simulink model "top_model_rw_desatTest"  (R2017b)
settings: Solver=FixedStepAuto  StartTime=0.0  StopTime=30000  FixedStep=.2  RelTol=1e-3  EnableMultiTasking=on
model workspace: external: MATLAB File C:\Users\Justin\Documents\00 MEng Project\PAN_ADCS\initialization\simulink_workspace_init.m (data not in the file)
undefined symbols (not defined in the file): h_init, hdmax, hmax, IAU, Imp_max, Imp_min, init, K_F, Kd, km, Kp, L_F, m_follower, match_tol, muE, ontime_max, ontime_min, q_init, s, Thrust_max, Thrust_min, wbn_init
libraries: aerolibtransform2 x12, aerolibconvert2 x8, sharedtransform x8, hEemethod x8, aerolibgravity2 x6, aerolibutil x6, aerolibcelestial x4, vrlib x4
(part 4 of 5)

== system top_model_rw_desatTest/Controller1/Normal Mode Control System/compute attitude error ==
  quat : Inport
  quat_cmd : Inport  Port=2
  Demux : Demux
  Demux1 : Demux
  Mux : Mux  Inputs=3
  Mux1 : Mux  Inputs=2
  Mux2 : Mux  Inputs=3
  Mux3 : Mux  Inputs=2
  Selector : Selector  InputPortWidth=4  IndexOptions=Index vector (dialog)  Indices=4  OutputSizes=1
  Switch : Switch
  quat_multiply (relative quat) : Subsystem
  quat_multiply (relative quat)1 : Subsystem
  reverse : Gain  Gain=-1  SaturateOnIntegerOverflow=on  OutDataTypeStr=Inherit: Same as input  ParamDataTypeStr=Inherit: Same as input
  reverse1 : Gain  Gain=-1  SaturateOnIntegerOverflow=on  OutDataTypeStr=Inherit: Same as input  ParamDataTypeStr=Inherit: Same as input
  quat error : Outport
  wires:
  Demux/1 -> Mux/1
  Demux/2 -> Mux/2
  Demux/3 -> Mux/3
  Mux/1 -> reverse/1
  Mux1/1 -> quat_multiply (relative quat)/2(q_ab)
  Demux/4 -> Mux1/2
  reverse/1 -> Mux1/1
  Mux3/1 -> quat_multiply (relative quat)1/2(q_ab)
  Demux1/1 -> Mux2/1
  Demux1/2 -> Mux2/2
  Demux1/3 -> Mux2/3
  quat_cmd/1 -> Demux1/1, Demux/1
  Mux2/1 -> Mux3/1
  quat/1 -> quat_multiply (relative quat)1/1(q_bc), quat_multiply (relative quat)/1(q_bc)
  Demux1/4 -> reverse1/1
  reverse1/1 -> Mux3/2
  quat_multiply (relative quat)1/1(q_ac) -> Switch/3
  quat_multiply (relative quat)/1(q_ac) -> Selector/1, Switch/1
  Switch/1 -> quat error/1
  Selector/1 -> Switch/2

== system top_model_rw_desatTest/Controller1/Propulsion/Enabled Subsystem ==
  In1 : Inport
  Enable : EnablePort
  Out1 : Outport
  wires:
  In1/1 -> Out1/1

== system top_model_rw_desatTest/Controller1/Propulsion/Subsystem ==
  hit : Inport
  ontime : Inport  Port=2
  "Thrust_vec " : Inport  Port=3
  Activation : Subsystem
  Constant1 : Constant  Value=[0;0;0]
  Subsystem : Subsystem
  Switch : Switch  Criteria=u2 > Threshold
  imp_cmd : Outport
  wires:
  Constant1/1 -> Switch/3
  ontime/1 -> Activation/2(T_maneuver)
  Subsystem/1(value) -> Switch/2
  "Thrust_vec "/1 -> Switch/1
  hit/1 -> Subsystem/1(input), Activation/1(hit)
  Activation/1(man_end) -> Subsystem/2(overwrite trigger)
  Switch/1 -> imp_cmd/1

== system top_model_rw_desatTest/Controller1/Propulsion/Subsystem1 ==
  input : Inport
  overwrite trigger : Inport  Port=2
  Data Store Memory : DataStoreMemory  DataStoreName=Mem  ShowAdditionalParam=off
  Data Store Read : DataStoreRead  DataStoreName=Mem  SampleTime=[0,0]  DataStoreElements=Mem
  Data Store Write : DataStoreWrite  DataStoreName=Mem  SampleTime=[0,0]  DataStoreElements=Mem
  Switch : Switch  Criteria=u2 > Threshold
  value : Outport
  wires:
  input/1 -> Switch/1
  Switch/1 -> value/1, Data Store Write/1
  Data Store Read/1 -> Switch/3
  overwrite trigger/1 -> Switch/2

== system top_model_rw_desatTest/Controller1/quat to DCM/Subsystem ==
  In1 : Inport
  3x3 : Reshape  OutputDimensionality=Customize  OutputDimensions=[3,3]
  Demux : Demux  Outputs=3
  Gain : Gain  Gain=-1  SaturateOnIntegerOverflow=on  OutDataTypeStr=Inherit: Same as input  ParamDataTypeStr=Inherit: Same as input
  Gain1 : Gain  Gain=-1  SaturateOnIntegerOverflow=on  OutDataTypeStr=Inherit: Same as input  ParamDataTypeStr=Inherit: Same as input
  Gain2 : Gain  Gain=-1  SaturateOnIntegerOverflow=on  OutDataTypeStr=Inherit: Same as input  ParamDataTypeStr=Inherit: Same as input
  Mux : Mux  Inputs=9
  "diag 0 " : Constant  Value=0
  Out1 : Outport
  wires:
  In1/1 -> Demux/1
  3x3/1 -> Out1/1
  "diag 0 "/1 -> Mux/1, Mux/5, Mux/9
  Mux/1 -> 3x3/1
  Demux/3 -> Mux/2, Gain1/1
  Gain/1 -> Mux/3
  Demux/2 -> Gain/1, Mux/7
  Gain1/1 -> Mux/4
  Demux/1 -> Mux/6, Gain2/1
  Gain2/1 -> Mux/8

== system top_model_rw_desatTest/FWR_Plant/Quaternion Integration/q_normalize ==
  q_in : Inport  PortDimensions=4
  Dot Product : DotProduct  InputSameDT=on  OutDataTypeStr=Inherit: Inherit via internal rule
  Math Function : Math  Operator=sqrt  SaturateOnIntegerOverflow=on
  Product : Product  Inputs=*/  SaturateOnIntegerOverflow=on  InputSameDT=on  OutDataTypeStr=Inherit: Same as first input
  q_out : Outport
  wires:
  q_in/1 -> Dot Product/1, Dot Product/2, Product/1
  Dot Product/1 -> Math Function/1
  Math Function/1 -> Product/2
  Product/1 -> q_out/1

== system top_model_rw_desatTest/FWR_Plant/Quaternion Integration/qderiv ==
  w : Inport
  q : Inport  Port=2
  Mux : Mux  Inputs=2
  Mux1 : Mux
  qd1 : Fcn  Expr=(u(7)*u(1)-u(6)*u(2)+u(5)*u(3))/2
  qd2 : Fcn  Expr=(u(6)*u(1)+u(7)*u(2)-u(4)*u(3))/2
  qd3 : Fcn  Expr=(-u(5)*u(1)+u(4)*u(2)+u(7)*u(3))/2
  qd4 : Fcn  Expr=(-u(4)*u(1)-u(5)*u(2)-u(6)*u(3))/2
  qd : Outport
  wires:
  w/1 -> Mux/1
  q/1 -> Mux/2
  Mux/1 -> qd3/1, qd4/1, qd1/1, qd2/1
  qd1/1 -> Mux1/1
  qd2/1 -> Mux1/2
  qd3/1 -> Mux1/3
  qd4/1 -> Mux1/4
  Mux1/1 -> qd/1

== system top_model_rw_desatTest/FWR_Sensor Model/quat to DCM/Subsystem ==
  In1 : Inport
  3x3 : Reshape  OutputDimensionality=Customize  OutputDimensions=[3,3]
  Demux : Demux  Outputs=3
  Gain : Gain  Gain=-1  SaturateOnIntegerOverflow=on  OutDataTypeStr=Inherit: Same as input  ParamDataTypeStr=Inherit: Same as input
  Gain1 : Gain  Gain=-1  SaturateOnIntegerOverflow=on  OutDataTypeStr=Inherit: Same as input  ParamDataTypeStr=Inherit: Same as input
  Gain2 : Gain  Gain=-1  SaturateOnIntegerOverflow=on  OutDataTypeStr=Inherit: Same as input  ParamDataTypeStr=Inherit: Same as input
  Mux : Mux  Inputs=9
  "diag 0 " : Constant  Value=0
  Out1 : Outport
  wires:
  In1/1 -> Demux/1
  3x3/1 -> Out1/1
  "diag 0 "/1 -> Mux/1, Mux/5, Mux/9
  Mux/1 -> 3x3/1
  Demux/3 -> Mux/2, Gain1/1
  Gain/1 -> Mux/3
  Demux/2 -> Gain/1, Mux/7
  Gain1/1 -> Mux/4
  Demux/1 -> Mux/6, Gain2/1
  Gain2/1 -> Mux/8

== system top_model_rw_desatTest/GNC/Follower Maneuver/Optimal Latitude Calc ==
  "r " : Inport
  "v " : Inport  Port=2
  muE : Inport  Port=3
  x_tgt : Inport  Port=4
  x_f : Inport  Port=5
  Update Trigger : Inport  Port=6
  Constant : Constant  Value=K_F
  Constant1 : Constant  Value=L_F
  Enabled Subsystem : Subsystem  TreatAsAtomicUnit=on
  dV_opt : Outport
  long_opt : Outport  Port=2
  pos_opt : Outport  Port=3
  wires:
  Enabled Subsystem/2(long_opt) -> long_opt/1
  "r "/1 -> Enabled Subsystem/1(r)
  "v "/1 -> Enabled Subsystem/2(v)
  muE/1 -> Enabled Subsystem/7("muE ")
  x_tgt/1 -> Enabled Subsystem/3(x_tgt)
  x_f/1 -> Enabled Subsystem/4(x_f)
  Constant/1 -> Enabled Subsystem/5(K)
  Constant1/1 -> Enabled Subsystem/6(L)
  Enabled Subsystem/1(dV_opt) -> dV_opt/1
  Enabled Subsystem/3(pos_opt) -> pos_opt/1
  Update Trigger/1 -> Enabled Subsystem/Enable

== system top_model_rw_desatTest/LDR_Plant/Quaternion Integration/q_normalize ==
  q_in : Inport  PortDimensions=4
  Dot Product : DotProduct  InputSameDT=on  OutDataTypeStr=Inherit: Inherit via internal rule
  Math Function : Math  Operator=sqrt  SaturateOnIntegerOverflow=on
  Product : Product  Inputs=*/  SaturateOnIntegerOverflow=on  InputSameDT=on  OutDataTypeStr=Inherit: Same as first input
  q_out : Outport
  wires:
  q_in/1 -> Dot Product/1, Dot Product/2, Product/1
  Dot Product/1 -> Math Function/1
  Math Function/1 -> Product/2
  Product/1 -> q_out/1

== system top_model_rw_desatTest/LDR_Plant/Quaternion Integration/qderiv ==
  w : Inport
  q : Inport  Port=2
  Mux : Mux  Inputs=2
  Mux1 : Mux
  qd1 : Fcn  Expr=(u(7)*u(1)-u(6)*u(2)+u(5)*u(3))/2
  qd2 : Fcn  Expr=(u(6)*u(1)+u(7)*u(2)-u(4)*u(3))/2
  qd3 : Fcn  Expr=(-u(5)*u(1)+u(4)*u(2)+u(7)*u(3))/2
  qd4 : Fcn  Expr=(-u(4)*u(1)-u(5)*u(2)-u(6)*u(3))/2
  qd : Outport
  wires:
  w/1 -> Mux/1
  q/1 -> Mux/2
  Mux/1 -> qd3/1, qd4/1, qd1/1, qd2/1
  qd1/1 -> Mux1/1
  qd2/1 -> Mux1/2
  qd3/1 -> Mux1/3
  qd4/1 -> Mux1/4
  Mux1/1 -> qd/1

== system top_model_rw_desatTest/LDR_Sensor Model/quat to DCM/Subsystem ==
  In1 : Inport
  3x3 : Reshape  OutputDimensionality=Customize  OutputDimensions=[3,3]
  Demux : Demux  Outputs=3
  Gain : Gain  Gain=-1  SaturateOnIntegerOverflow=on  OutDataTypeStr=Inherit: Same as input  ParamDataTypeStr=Inherit: Same as input
  Gain1 : Gain  Gain=-1  SaturateOnIntegerOverflow=on  OutDataTypeStr=Inherit: Same as input  ParamDataTypeStr=Inherit: Same as input
  Gain2 : Gain  Gain=-1  SaturateOnIntegerOverflow=on  OutDataTypeStr=Inherit: Same as input  ParamDataTypeStr=Inherit: Same as input
  Mux : Mux  Inputs=9
  "diag 0 " : Constant  Value=0
  Out1 : Outport
  wires:
  In1/1 -> Demux/1
  3x3/1 -> Out1/1
  "diag 0 "/1 -> Mux/1, Mux/5, Mux/9
  Mux/1 -> 3x3/1
  Demux/3 -> Mux/2, Gain1/1
  Gain/1 -> Mux/3
  Demux/2 -> Gain/1, Mux/7
  Gain1/1 -> Mux/4
  Demux/1 -> Mux/6, Gain2/1
  Gain2/1 -> Mux/8

== system top_model_rw_desatTest/Actuator Model/Rigid Body with Momentum Actuators and energy dissipation/quat to DCM/Subsystem ==
  In1 : Inport
  3x3 : Reshape  OutputDimensionality=Customize  OutputDimensions=[3,3]
  Demux : Demux  Outputs=3
  Gain : Gain  Gain=-1  SaturateOnIntegerOverflow=on  OutDataTypeStr=Inherit: Same as input  ParamDataTypeStr=Inherit: Same as input
  Gain1 : Gain  Gain=-1  SaturateOnIntegerOverflow=on  OutDataTypeStr=Inherit: Same as input  ParamDataTypeStr=Inherit: Same as input
  Gain2 : Gain  Gain=-1  SaturateOnIntegerOverflow=on  OutDataTypeStr=Inherit: Same as input  ParamDataTypeStr=Inherit: Same as input
  Mux : Mux  Inputs=9
  "diag 0 " : Constant  Value=0
  Out1 : Outport
  wires:
  Gain2/1 -> Mux/8
  Demux/1 -> Gain2/1, Mux/6
  Gain1/1 -> Mux/4
  Demux/2 -> Mux/7, Gain/1
  Gain/1 -> Mux/3
  Demux/3 -> Gain1/1, Mux/2
  Mux/1 -> 3x3/1
  "diag 0 "/1 -> Mux/9, Mux/5, Mux/1
  3x3/1 -> Out1/1
  In1/1 -> Demux/1

== system top_model_rw_desatTest/Actuator Model/Rigid Body with Momentum Actuators and energy dissipation/quat to DCM1/Subsystem ==
  In1 : Inport
  3x3 : Reshape  OutputDimensionality=Customize  OutputDimensions=[3,3]
  Demux : Demux  Outputs=3
  Gain : Gain  Gain=-1  SaturateOnIntegerOverflow=on  OutDataTypeStr=Inherit: Same as input  ParamDataTypeStr=Inherit: Same as input
  Gain1 : Gain  Gain=-1  SaturateOnIntegerOverflow=on  OutDataTypeStr=Inherit: Same as input  ParamDataTypeStr=Inherit: Same as input
  Gain2 : Gain  Gain=-1  SaturateOnIntegerOverflow=on  OutDataTypeStr=Inherit: Same as input  ParamDataTypeStr=Inherit: Same as input
  Mux : Mux  Inputs=9
  "diag 0 " : Constant  Value=0
  Out1 : Outport
  wires:
  Gain2/1 -> Mux/8
  Demux/1 -> Gain2/1, Mux/6
  Gain1/1 -> Mux/4
  Demux/2 -> Mux/7, Gain/1
  Gain/1 -> Mux/3
  Demux/3 -> Gain1/1, Mux/2
  Mux/1 -> 3x3/1
  "diag 0 "/1 -> Mux/9, Mux/5, Mux/1
  3x3/1 -> Out1/1
  In1/1 -> Demux/1

== system top_model_rw_desatTest/Actuator Model1/Rigid Body with Momentum Actuators and energy dissipation/quat to DCM/Subsystem ==
  In1 : Inport
  3x3 : Reshape  OutputDimensionality=Customize  OutputDimensions=[3,3]
  Demux : Demux  Outputs=3
  Gain : Gain  Gain=-1  SaturateOnIntegerOverflow=on  OutDataTypeStr=Inherit: Same as input  ParamDataTypeStr=Inherit: Same as input
  Gain1 : Gain  Gain=-1  SaturateOnIntegerOverflow=on  OutDataTypeStr=Inherit: Same as input  ParamDataTypeStr=Inherit: Same as input
  Gain2 : Gain  Gain=-1  SaturateOnIntegerOverflow=on  OutDataTypeStr=Inherit: Same as input  ParamDataTypeStr=Inherit: Same as input
  Mux : Mux  Inputs=9
  "diag 0 " : Constant  Value=0
  Out1 : Outport
  wires:
  Gain2/1 -> Mux/8
  Demux/1 -> Gain2/1, Mux/6
  Gain1/1 -> Mux/4
  Demux/2 -> Mux/7, Gain/1
  Gain/1 -> Mux/3
  Demux/3 -> Gain1/1, Mux/2
  Mux/1 -> 3x3/1
  "diag 0 "/1 -> Mux/9, Mux/5, Mux/1
  3x3/1 -> Out1/1
  In1/1 -> Demux/1

== system top_model_rw_desatTest/Actuator Model1/Rigid Body with Momentum Actuators and energy dissipation/quat to DCM1/Subsystem ==
  In1 : Inport
  3x3 : Reshape  OutputDimensionality=Customize  OutputDimensions=[3,3]
  Demux : Demux  Outputs=3
  Gain : Gain  Gain=-1  SaturateOnIntegerOverflow=on  OutDataTypeStr=Inherit: Same as input  ParamDataTypeStr=Inherit: Same as input
  Gain1 : Gain  Gain=-1  SaturateOnIntegerOverflow=on  OutDataTypeStr=Inherit: Same as input  ParamDataTypeStr=Inherit: Same as input
  Gain2 : Gain  Gain=-1  SaturateOnIntegerOverflow=on  OutDataTypeStr=Inherit: Same as input  ParamDataTypeStr=Inherit: Same as input
  Mux : Mux  Inputs=9
  "diag 0 " : Constant  Value=0
  Out1 : Outport
  wires:
  Gain2/1 -> Mux/8
  Demux/1 -> Gain2/1, Mux/6
  Gain1/1 -> Mux/4
  Demux/2 -> Mux/7, Gain/1
  Gain/1 -> Mux/3
  Demux/3 -> Gain1/1, Mux/2
  Mux/1 -> 3x3/1
  "diag 0 "/1 -> Mux/9, Mux/5, Mux/1
  3x3/1 -> Out1/1
  In1/1 -> Demux/1

== system top_model_rw_desatTest/Attitude Determination and Desired Attitude/Attitude Determination/Generate reference vectors from Ephemeris and Magnetic Field Model/DecimalYearIncrement ==
  note: day
  clock_sec : Inport
  Add : Sum
  Constant : Constant  Value=init.year
  Constant1 : Constant  Value=init.month
  Constant2 : Constant  Value=init.day
  Constant3 : Constant  Value=init.hour
  Constant4 : Constant  Value=init.min
  Constant5 : Constant  Value=init.min
  Divide : Product  Inputs=*/
  MATLAB Function : MATLAB Function  TreatAsAtomicUnit=on
  Product2 : Product  Inputs=*/
  day2decimalYear : Constant  Value=365
  sec2day : Constant  Value=86400
  DecimalYear : Outport
  wires:
  Product2/1 -> Divide/1
  sec2day/1 -> Product2/2
  Add/1 -> DecimalYear/1
  Constant3/1 -> MATLAB Function/4(hour)
  day2decimalYear/1 -> Divide/2
  Divide/1 -> Add/1
  MATLAB Function/1(DecimalYear) -> Add/2
  Constant1/1 -> MATLAB Function/2(month)
  Constant/1 -> MATLAB Function/1(year)
  Constant4/1 -> MATLAB Function/5(minute)
  Constant5/1 -> MATLAB Function/6(second)
  clock_sec/1 -> Product2/1
  Constant2/1 -> MATLAB Function/3(day)

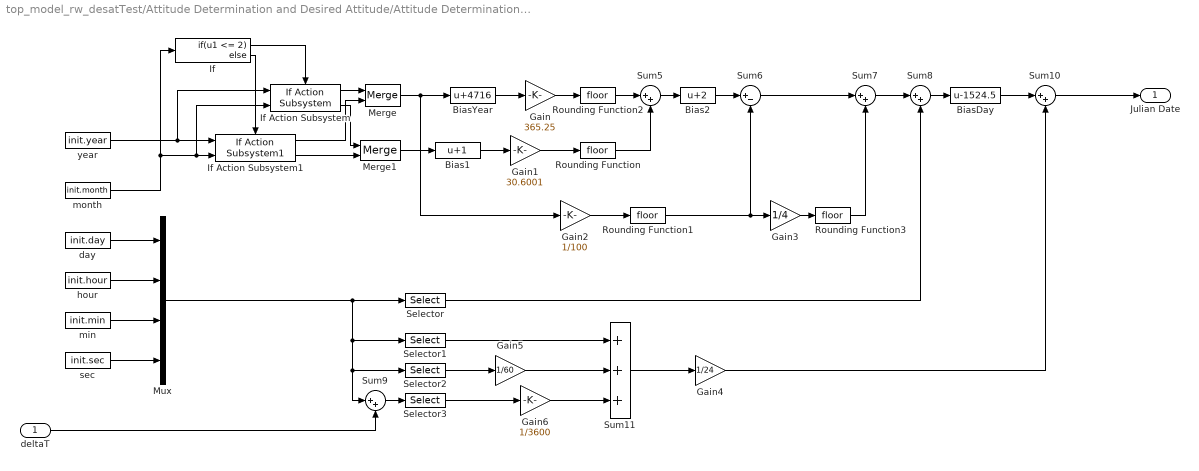
== system top_model_rw_desatTest/Attitude Determination and Desired Attitude/Attitude Determination/Generate reference vectors from Ephemeris and Magnetic Field Model/Julian Date ==
  deltaT : Inport  OutMin=0  PortDimensions=1
  Bias1 : Bias  Bias=1
  Bias2 : Bias  Bias=2
  BiasDay : Bias  Bias=-1524.5
  BiasYear : Bias  Bias=4716
  Gain : Gain  Gain=365.25
  Gain1 : Gain  Gain=30.6001
  Gain2 : Gain  Gain=1/100
  Gain3 : Gain  Gain=1/4
  Gain4 : Gain  Gain=1/24
  Gain5 : Gain  Gain=1/60
  Gain6 : Gain  Gain=1/3600
  If : If  IfExpression=u1 <= 2
  If Action Subsystem : aerolibconvert2/Julian Date Conversion/If Action Subsystem
      settings: SourceProductName=Aerospace Blockset  SourceProductBaseCode=AE
  If Action Subsystem1 : aerolibconvert2/Julian Date Conversion/If Action Subsystem1
      settings: SourceProductName=Aerospace Blockset  SourceProductBaseCode=AE
  Merge : Merge
  Merge1 : Merge
  Mux : Mux
  Rounding Function{,1..3} (4 alike) : Rounding
  Selector : Selector  InputPortWidth=4  IndexOptions=Index vector (dialog)  Indices=[1]  OutputSizes=1
  Selector1 : Selector  InputPortWidth=4  IndexOptions=Index vector (dialog)  Indices=[2]  OutputSizes=1
  Selector2 : Selector  InputPortWidth=4  IndexOptions=Index vector (dialog)  Indices=[3]  OutputSizes=1
  Selector3 : Selector  InputPortWidth=4  IndexOptions=Index vector (dialog)  Indices=[4]  OutputSizes=1
  Sum{5,7..10} (5 alike) : Sum  Inputs=|++
  Sum11 : Sum  Inputs=+++
  Sum6 : Sum  Inputs=|+-
  day : Constant  Value=init.day
  hour : Constant  Value=init.hour
  min : Constant  Value=init.min
  month : Constant  Value=init.month
  sec : Constant  Value=init.sec
  year : Constant  Value=init.year
  Julian Date : Outport
  wires:
  If Action Subsystem/1 -> Merge/1
  If/2 -> If Action Subsystem1/Action
  year/1 -> If Action Subsystem/1, If Action Subsystem1/1
  If/1 -> If Action Subsystem/Action
  If Action Subsystem/2 -> Merge1/1
  Rounding Function3/1 -> Sum7/2
  deltaT/1 -> Sum9/2
  day/1 -> Mux/1
  Merge1/1 -> Bias1/1
  Gain/1 -> Rounding Function2/1
  Gain2/1 -> Rounding Function1/1
  Merge/1 -> Gain2/1, BiasYear/1
  Selector3/1 -> Gain6/1
  Sum6/1 -> Sum7/1
  Gain5/1 -> Sum11/2
  BiasYear/1 -> Gain/1
  Selector2/1 -> Gain5/1
  Gain6/1 -> Sum11/3
  Sum11/1 -> Gain4/1
  Gain3/1 -> Rounding Function3/1
  Selector1/1 -> Sum11/1
  If Action Subsystem1/1 -> Merge/2
  Sum7/1 -> Sum8/1
  Mux/1 -> Selector1/1, Sum9/1, Selector2/1, Selector/1
  Sum10/1 -> Julian Date/1
  Selector/1 -> Sum8/2
  Bias1/1 -> Gain1/1
  sec/1 -> Mux/4
  If Action Subsystem1/2 -> Merge1/2
  Sum5/1 -> Bias2/1
  BiasDay/1 -> Sum10/1
  Gain1/1 -> Rounding Function/1
  Rounding Function1/1 -> Gain3/1, Sum6/2
  Bias2/1 -> Sum6/1
  Sum8/1 -> BiasDay/1
  Rounding Function2/1 -> Sum5/1
  Rounding Function/1 -> Sum5/2
  month/1 -> If Action Subsystem/2, If Action Subsystem1/2, If/1
  min/1 -> Mux/3
  hour/1 -> Mux/2
  Gain4/1 -> Sum10/2
  Sum9/1 -> Selector3/1

== system top_model_rw_desatTest/Attitude Determination and Desired Attitude/Position and Velocity to Desired Attitude in Quat/CreateDCM_be/normalize ==
  r : Inport
  Dot Product : DotProduct  InputSameDT=on  OutDataTypeStr=Inherit: Inherit via internal rule
  Math Function : Math  Operator=sqrt  SaturateOnIntegerOverflow=on
  Product : Product  Inputs=*/  SaturateOnIntegerOverflow=on  InputSameDT=on  OutDataTypeStr=Inherit: Same as first input
  r_hat : Outport
  wires:
  r/1 -> Dot Product/1, Dot Product/2, Product/1
  Dot Product/1 -> Math Function/1
  Math Function/1 -> Product/2
  Product/1 -> r_hat/1

== system top_model_rw_desatTest/Attitude Determination and Desired Attitude/Position and Velocity to Desired Attitude in Quat/CreateDCM_be/normalize2 ==
  v : Inport
  Dot Product : DotProduct  InputSameDT=on  OutDataTypeStr=Inherit: Inherit via internal rule
  Math Function : Math  Operator=sqrt  SaturateOnIntegerOverflow=on
  Product : Product  Inputs=*/  SaturateOnIntegerOverflow=on  InputSameDT=on  OutDataTypeStr=Inherit: Same as first input
  v_hat : Outport
  wires:
  v/1 -> Dot Product/1, Dot Product/2, Product/1
  Dot Product/1 -> Math Function/1
  Math Function/1 -> Product/2
  Product/1 -> v_hat/1

== system top_model_rw_desatTest/Attitude Determination and Desired Attitude/Position and Velocity to Desired Attitude in Quat/quat to DCM/Subsystem ==
  In1 : Inport
  3x3 : Reshape  OutputDimensionality=Customize  OutputDimensions=[3,3]
  Demux : Demux  Outputs=3
  Gain : Gain  Gain=-1  SaturateOnIntegerOverflow=on  OutDataTypeStr=Inherit: Same as input  ParamDataTypeStr=Inherit: Same as input
  Gain1 : Gain  Gain=-1  SaturateOnIntegerOverflow=on  OutDataTypeStr=Inherit: Same as input  ParamDataTypeStr=Inherit: Same as input
  Gain2 : Gain  Gain=-1  SaturateOnIntegerOverflow=on  OutDataTypeStr=Inherit: Same as input  ParamDataTypeStr=Inherit: Same as input
  Mux : Mux  Inputs=9
  "diag 0 " : Constant  Value=0
  Out1 : Outport
  wires:
  Gain2/1 -> Mux/8
  Demux/1 -> Gain2/1, Mux/6
  Gain1/1 -> Mux/4
  Demux/2 -> Mux/7, Gain/1
  Gain/1 -> Mux/3
  Demux/3 -> Gain1/1, Mux/2
  Mux/1 -> 3x3/1
  "diag 0 "/1 -> Mux/9, Mux/5, Mux/1
  3x3/1 -> Out1/1
  In1/1 -> Demux/1

== system top_model_rw_desatTest/Attitude Determination and Desired Attitude1/Attitude Determination/Generate reference vectors from Ephemeris and Magnetic Field Model/DecimalYearIncrement ==
  note: day
  clock_sec : Inport
  Add : Sum
  Constant : Constant  Value=init.year
  Constant1 : Constant  Value=init.month
  Constant2 : Constant  Value=init.day
  Constant3 : Constant  Value=init.hour
  Constant4 : Constant  Value=init.min
  Constant5 : Constant  Value=init.min
  Divide : Product  Inputs=*/
  MATLAB Function : MATLAB Function  TreatAsAtomicUnit=on
  Product2 : Product  Inputs=*/
  day2decimalYear : Constant  Value=365
  sec2day : Constant  Value=86400
  DecimalYear : Outport
  wires:
  Product2/1 -> Divide/1
  sec2day/1 -> Product2/2
  Add/1 -> DecimalYear/1
  Constant3/1 -> MATLAB Function/4(hour)
  day2decimalYear/1 -> Divide/2
  Divide/1 -> Add/1
  MATLAB Function/1(DecimalYear) -> Add/2
  Constant1/1 -> MATLAB Function/2(month)
  Constant/1 -> MATLAB Function/1(year)
  Constant4/1 -> MATLAB Function/5(minute)
  Constant5/1 -> MATLAB Function/6(second)
  clock_sec/1 -> Product2/1
  Constant2/1 -> MATLAB Function/3(day)

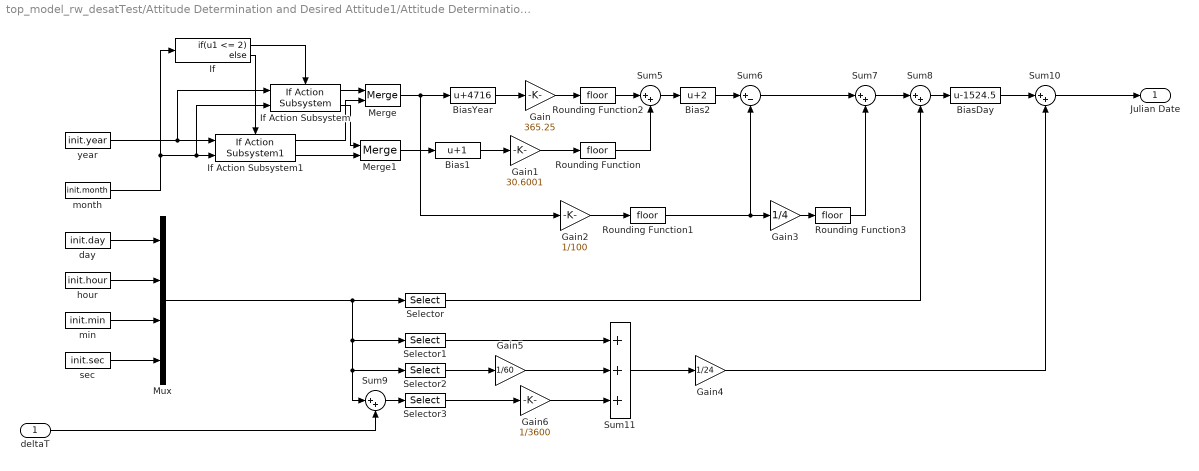
== system top_model_rw_desatTest/Attitude Determination and Desired Attitude1/Attitude Determination/Generate reference vectors from Ephemeris and Magnetic Field Model/Julian Date ==
  deltaT : Inport  OutMin=0  PortDimensions=1
  Bias1 : Bias  Bias=1
  Bias2 : Bias  Bias=2
  BiasDay : Bias  Bias=-1524.5
  BiasYear : Bias  Bias=4716
  Gain : Gain  Gain=365.25
  Gain1 : Gain  Gain=30.6001
  Gain2 : Gain  Gain=1/100
  Gain3 : Gain  Gain=1/4
  Gain4 : Gain  Gain=1/24
  Gain5 : Gain  Gain=1/60
  Gain6 : Gain  Gain=1/3600
  If : If  IfExpression=u1 <= 2
  If Action Subsystem : aerolibconvert2/Julian Date Conversion/If Action Subsystem
      settings: SourceProductName=Aerospace Blockset  SourceProductBaseCode=AE
  If Action Subsystem1 : aerolibconvert2/Julian Date Conversion/If Action Subsystem1
      settings: SourceProductName=Aerospace Blockset  SourceProductBaseCode=AE
  Merge : Merge
  Merge1 : Merge
  Mux : Mux
  Rounding Function{,1..3} (4 alike) : Rounding
  Selector : Selector  InputPortWidth=4  IndexOptions=Index vector (dialog)  Indices=[1]  OutputSizes=1
  Selector1 : Selector  InputPortWidth=4  IndexOptions=Index vector (dialog)  Indices=[2]  OutputSizes=1
  Selector2 : Selector  InputPortWidth=4  IndexOptions=Index vector (dialog)  Indices=[3]  OutputSizes=1
  Selector3 : Selector  InputPortWidth=4  IndexOptions=Index vector (dialog)  Indices=[4]  OutputSizes=1
  Sum{5,7..10} (5 alike) : Sum  Inputs=|++
  Sum11 : Sum  Inputs=+++
  Sum6 : Sum  Inputs=|+-
  day : Constant  Value=init.day
  hour : Constant  Value=init.hour
  min : Constant  Value=init.min
  month : Constant  Value=init.month
  sec : Constant  Value=init.sec
  year : Constant  Value=init.year
  Julian Date : Outport
  wires:
  If Action Subsystem/1 -> Merge/1
  If/2 -> If Action Subsystem1/Action
  year/1 -> If Action Subsystem/1, If Action Subsystem1/1
  If/1 -> If Action Subsystem/Action
  If Action Subsystem/2 -> Merge1/1
  Rounding Function3/1 -> Sum7/2
  deltaT/1 -> Sum9/2
  day/1 -> Mux/1
  Merge1/1 -> Bias1/1
  Gain/1 -> Rounding Function2/1
  Gain2/1 -> Rounding Function1/1
  Merge/1 -> Gain2/1, BiasYear/1
  Selector3/1 -> Gain6/1
  Sum6/1 -> Sum7/1
  Gain5/1 -> Sum11/2
  BiasYear/1 -> Gain/1
  Selector2/1 -> Gain5/1
  Gain6/1 -> Sum11/3
  Sum11/1 -> Gain4/1
  Gain3/1 -> Rounding Function3/1
  Selector1/1 -> Sum11/1
  If Action Subsystem1/1 -> Merge/2
  Sum7/1 -> Sum8/1
  Mux/1 -> Selector1/1, Sum9/1, Selector2/1, Selector/1
  Sum10/1 -> Julian Date/1
  Selector/1 -> Sum8/2
  Bias1/1 -> Gain1/1
  sec/1 -> Mux/4
  If Action Subsystem1/2 -> Merge1/2
  Sum5/1 -> Bias2/1
  BiasDay/1 -> Sum10/1
  Gain1/1 -> Rounding Function/1
  Rounding Function1/1 -> Gain3/1, Sum6/2
  Bias2/1 -> Sum6/1
  Sum8/1 -> BiasDay/1
  Rounding Function2/1 -> Sum5/1
  Rounding Function/1 -> Sum5/2
  month/1 -> If Action Subsystem/2, If Action Subsystem1/2, If/1
  min/1 -> Mux/3
  hour/1 -> Mux/2
  Gain4/1 -> Sum10/2
  Sum9/1 -> Selector3/1

== system top_model_rw_desatTest/Attitude Determination and Desired Attitude1/Position and Velocity to Desired Attitude in Quat/CreateDCM_be/normalize ==
  r : Inport
  Dot Product : DotProduct  InputSameDT=on  OutDataTypeStr=Inherit: Inherit via internal rule
  Math Function : Math  Operator=sqrt  SaturateOnIntegerOverflow=on
  Product : Product  Inputs=*/  SaturateOnIntegerOverflow=on  InputSameDT=on  OutDataTypeStr=Inherit: Same as first input
  r_hat : Outport
  wires:
  r/1 -> Dot Product/1, Dot Product/2, Product/1
  Dot Product/1 -> Math Function/1
  Math Function/1 -> Product/2
  Product/1 -> r_hat/1

== system top_model_rw_desatTest/Attitude Determination and Desired Attitude1/Position and Velocity to Desired Attitude in Quat/CreateDCM_be/normalize2 ==
  v : Inport
  Dot Product : DotProduct  InputSameDT=on  OutDataTypeStr=Inherit: Inherit via internal rule
  Math Function : Math  Operator=sqrt  SaturateOnIntegerOverflow=on
  Product : Product  Inputs=*/  SaturateOnIntegerOverflow=on  InputSameDT=on  OutDataTypeStr=Inherit: Same as first input
  v_hat : Outport
  wires:
  v/1 -> Dot Product/1, Dot Product/2, Product/1
  Dot Product/1 -> Math Function/1
  Math Function/1 -> Product/2
  Product/1 -> v_hat/1

== system top_model_rw_desatTest/Attitude Determination and Desired Attitude1/Position and Velocity to Desired Attitude in Quat/quat to DCM/Subsystem ==
  In1 : Inport
  3x3 : Reshape  OutputDimensionality=Customize  OutputDimensions=[3,3]
  Demux : Demux  Outputs=3
  Gain : Gain  Gain=-1  SaturateOnIntegerOverflow=on  OutDataTypeStr=Inherit: Same as input  ParamDataTypeStr=Inherit: Same as input
  Gain1 : Gain  Gain=-1  SaturateOnIntegerOverflow=on  OutDataTypeStr=Inherit: Same as input  ParamDataTypeStr=Inherit: Same as input
  Gain2 : Gain  Gain=-1  SaturateOnIntegerOverflow=on  OutDataTypeStr=Inherit: Same as input  ParamDataTypeStr=Inherit: Same as input
  Mux : Mux  Inputs=9
  "diag 0 " : Constant  Value=0
  Out1 : Outport
  wires:
  Gain2/1 -> Mux/8
  Demux/1 -> Gain2/1, Mux/6
  Gain1/1 -> Mux/4
  Demux/2 -> Mux/7, Gain/1
  Gain/1 -> Mux/3
  Demux/3 -> Gain1/1, Mux/2
  Mux/1 -> 3x3/1
  "diag 0 "/1 -> Mux/9, Mux/5, Mux/1
  3x3/1 -> Out1/1
  In1/1 -> Demux/1

== system top_model_rw_desatTest/Controller/Free Rigid Body with Momentum Actuators2/Quaternion Integration/q_normalize ==
  q_in : Inport  PortDimensions=4
  Dot Product : DotProduct  InputSameDT=on  OutDataTypeStr=Inherit: Inherit via internal rule
  Math Function : Math  Operator=sqrt  SaturateOnIntegerOverflow=on
  Product : Product  Inputs=*/  SaturateOnIntegerOverflow=on  InputSameDT=on  OutDataTypeStr=Inherit: Same as first input
  q_out : Outport
  wires:
  q_in/1 -> Dot Product/1, Dot Product/2, Product/1
  Dot Product/1 -> Math Function/1
  Math Function/1 -> Product/2
  Product/1 -> q_out/1

== system top_model_rw_desatTest/Controller/Free Rigid Body with Momentum Actuators2/Quaternion Integration/qderiv ==
  w : Inport
  q : Inport  Port=2
  Mux : Mux  Inputs=2
  Mux1 : Mux
  qd1 : Fcn  Expr=(u(7)*u(1)-u(6)*u(2)+u(5)*u(3))/2
  qd2 : Fcn  Expr=(u(6)*u(1)+u(7)*u(2)-u(4)*u(3))/2
  qd3 : Fcn  Expr=(-u(5)*u(1)+u(4)*u(2)+u(7)*u(3))/2
  qd4 : Fcn  Expr=(-u(4)*u(1)-u(5)*u(2)-u(6)*u(3))/2
  qd : Outport
  wires:
  w/1 -> Mux/1
  q/1 -> Mux/2
  Mux/1 -> qd3/1, qd4/1, qd1/1, qd2/1
  qd1/1 -> Mux1/1
  qd2/1 -> Mux1/2
  qd3/1 -> Mux1/3
  qd4/1 -> Mux1/4
  Mux1/1 -> qd/1

== system top_model_rw_desatTest/Controller/Free Rigid Body with Momentum Actuators2/RWA Saturation Model (Maxon EC 32 Flat 15W 24V)/max rate check ==
  wheel h : Inport
  wheel hb : Inport  Port=2
  0 to 1 : Constant  Value=0  VectorParams1D=off
  "0 to 1 " : Constant  Value=0  VectorParams1D=off
  "0 to 1  " : Constant  Value=0  VectorParams1D=off
  Abs : Abs  SaturateOnIntegerOverflow=on
  Demux : Demux  Outputs=3
  Demux1 : Demux  Outputs=3
  Demux2 : Demux  Outputs=3
  Logical Operator : Logic
  Logical Operator1 : Logic
  Logical Operator2 : Logic
  Mux : Mux  Inputs=3
  Product : Product  SaturateOnIntegerOverflow=on  InputSameDT=on  OutDataTypeStr=Inherit: Same as first input
  Product1 : Product  SaturateOnIntegerOverflow=on  InputSameDT=on  OutDataTypeStr=Inherit: Same as first input
  Product2 : Product  SaturateOnIntegerOverflow=on  InputSameDT=on  OutDataTypeStr=Inherit: Same as first input
  Relational Operator : RelationalOperator  RndMeth=Nearest  InputSameDT=on
  Relational Operator1 : RelationalOperator  RndMeth=Nearest  InputSameDT=on
  Relational Operator2 : RelationalOperator  RndMeth=Nearest  InputSameDT=on
  Sign{,1..5} (6 alike) : Signum
  gt : RelationalOperator  Operator=>  RndMeth=Nearest  InputSameDT=on
  "gt " : RelationalOperator  Operator=>  RndMeth=Nearest  InputSameDT=on
  "gt  " : RelationalOperator  Operator=>  RndMeth=Nearest  InputSameDT=on
  hmax : Constant  Value=hmax  VectorParams1D=off
  hmax1 : Constant  Value=hmax  VectorParams1D=off
  hmax2 : Constant  Value=hmax  VectorParams1D=off
  saturated? : Outport
  wires:
  Abs/1 -> Demux/1
  Demux/1 -> Relational Operator/1
  Demux/2 -> Relational Operator1/1
  Demux/3 -> Relational Operator2/1
  hmax/1 -> Relational Operator/2
  hmax1/1 -> Relational Operator1/2
  hmax2/1 -> Relational Operator2/2
  wheel h/1 -> Abs/1, Demux2/1
  Mux/1 -> saturated?/1
  wheel hb/1 -> Demux1/1
  Demux1/1 -> Sign3/1
  Demux1/2 -> Sign4/1
  Demux1/3 -> Sign5/1
  Sign/1 -> Product/1
  Sign3/1 -> Product/2
  Sign1/1 -> Product1/1
  Sign4/1 -> Product1/2
  Sign2/1 -> Product2/1
  Sign5/1 -> Product2/2
  0 to 1/1 -> gt/2
  Product/1 -> gt/1
  "0 to 1 "/1 -> "gt "/2
  Product1/1 -> "gt "/1
  "0 to 1  "/1 -> "gt  "/2
  Product2/1 -> "gt  "/1
  Logical Operator/1 -> Mux/1
  Logical Operator1/1 -> Mux/2
  Logical Operator2/1 -> Mux/3
  Relational Operator/1 -> Logical Operator/1
  Relational Operator1/1 -> Logical Operator1/1
  Relational Operator2/1 -> Logical Operator2/1
  gt/1 -> Logical Operator/2
  "gt "/1 -> Logical Operator1/2
  "gt  "/1 -> Logical Operator2/2
  Demux2/1 -> Sign/1
  Demux2/2 -> Sign1/1
  Demux2/3 -> Sign2/1

== system top_model_rw_desatTest/Controller/Free Rigid Body with Momentum Actuators2/compute attitude error/quat_multiply (relative quat) ==
  q_bc : Inport
  q_ab : Inport  Port=2
  Mux : Mux  Inputs=2
  Mux1 : Mux
  qerr1 : Fcn  Expr=u(4)*u(5)+u(3)*u(6)-u(2)*u(7)+u(1)*u(8)
  qerr2 : Fcn  Expr=-u(3)*u(5)+u(4)*u(6)+u(1)*u(7)+u(2)*u(8)
  qerr3 : Fcn  Expr=u(2)*u(5)-u(1)*u(6)+u(4)*u(7)+u(3)*u(8)
  qerr4 : Fcn  Expr=-u(1)*u(5)-u(2)*u(6)-u(3)*u(7)+u(4)*u(8)
  q_ac : Outport
  wires:
  Mux1/1 -> q_ac/1
  qerr4/1 -> Mux1/4
  qerr3/1 -> Mux1/3
  qerr2/1 -> Mux1/2
  qerr1/1 -> Mux1/1
  Mux/1 -> qerr4/1, qerr3/1, qerr2/1, qerr1/1
  q_ab/1 -> Mux/2
  q_bc/1 -> Mux/1

== system top_model_rw_desatTest/Controller/Normal Mode Control System/compute attitude error/quat_multiply (relative quat) ==
  q_bc : Inport
  q_ab : Inport  Port=2
  Mux : Mux  Inputs=2
  Mux1 : Mux
  qerr1 : Fcn  Expr=u(4)*u(5)+u(3)*u(6)-u(2)*u(7)+u(1)*u(8)
  qerr2 : Fcn  Expr=-u(3)*u(5)+u(4)*u(6)+u(1)*u(7)+u(2)*u(8)
  qerr3 : Fcn  Expr=u(2)*u(5)-u(1)*u(6)+u(4)*u(7)+u(3)*u(8)
  qerr4 : Fcn  Expr=-u(1)*u(5)-u(2)*u(6)-u(3)*u(7)+u(4)*u(8)
  q_ac : Outport
  wires:
  Mux1/1 -> q_ac/1
  qerr4/1 -> Mux1/4
  qerr3/1 -> Mux1/3
  qerr2/1 -> Mux1/2
  qerr1/1 -> Mux1/1
  Mux/1 -> qerr4/1, qerr3/1, qerr2/1, qerr1/1
  q_ab/1 -> Mux/2
  q_bc/1 -> Mux/1

== system top_model_rw_desatTest/Controller/Normal Mode Control System/compute attitude error/quat_multiply (relative quat)1 ==
  q_bc : Inport
  q_ab : Inport  Port=2
  Mux : Mux  Inputs=2
  Mux1 : Mux
  qerr1 : Fcn  Expr=u(4)*u(5)+u(3)*u(6)-u(2)*u(7)+u(1)*u(8)
  qerr2 : Fcn  Expr=-u(3)*u(5)+u(4)*u(6)+u(1)*u(7)+u(2)*u(8)
  qerr3 : Fcn  Expr=u(2)*u(5)-u(1)*u(6)+u(4)*u(7)+u(3)*u(8)
  qerr4 : Fcn  Expr=-u(1)*u(5)-u(2)*u(6)-u(3)*u(7)+u(4)*u(8)
  q_ac : Outport
  wires:
  Mux1/1 -> q_ac/1
  qerr4/1 -> Mux1/4
  qerr3/1 -> Mux1/3
  qerr2/1 -> Mux1/2
  qerr1/1 -> Mux1/1
  Mux/1 -> qerr4/1, qerr3/1, qerr2/1, qerr1/1
  q_ab/1 -> Mux/2
  q_bc/1 -> Mux/1

== system top_model_rw_desatTest/Controller/Propulsion/Subsystem/Activation ==
  note: current time
  note: time of trigger
  note: t_trig + onTime
  hit : Inport
  T_maneuver : Inport  Port=2
  Add : Sum
  Clock : Clock
  Hit Crossing : HitCross
  Subsystem : Subsystem
  Subtract : Sum  Inputs=+-
  man_end : Outport
  wires:
  Clock/1 -> Subsystem/1(input), Subtract/1
  hit/1 -> Subsystem/2(overwrite trigger)
  Hit Crossing/1 -> man_end/1
  T_maneuver/1 -> Add/2
  Subsystem/1(value) -> Add/1
  Add/1 -> Subtract/2
  Subtract/1 -> Hit Crossing/1

== system top_model_rw_desatTest/Controller/Propulsion/Subsystem/Subsystem ==
  input : Inport
  overwrite trigger : Inport  Port=2
  Data Store Memory : DataStoreMemory  DataStoreName=Mem  ShowAdditionalParam=off
  Data Store Read : DataStoreRead  DataStoreName=Mem  SampleTime=[0,0]  DataStoreElements=Mem
  Data Store Write : DataStoreWrite  DataStoreName=Mem  SampleTime=[0,0]  DataStoreElements=Mem
  Switch : Switch  Criteria=u2 > Threshold
  value : Outport
  wires:
  input/1 -> Switch/1
  Switch/1 -> Data Store Write/1, value/1
  Data Store Read/1 -> Switch/3
  overwrite trigger/1 -> Switch/2

== system top_model_rw_desatTest/Controller1/Free Rigid Body with Momentum Actuators2/Quaternion Integration/q_normalize ==
  q_in : Inport  PortDimensions=4
  Dot Product : DotProduct  InputSameDT=on  OutDataTypeStr=Inherit: Inherit via internal rule
  Math Function : Math  Operator=sqrt  SaturateOnIntegerOverflow=on
  Product : Product  Inputs=*/  SaturateOnIntegerOverflow=on  InputSameDT=on  OutDataTypeStr=Inherit: Same as first input
  q_out : Outport
  wires:
  q_in/1 -> Dot Product/1, Dot Product/2, Product/1
  Dot Product/1 -> Math Function/1
  Math Function/1 -> Product/2
  Product/1 -> q_out/1

== system top_model_rw_desatTest/Controller1/Free Rigid Body with Momentum Actuators2/Quaternion Integration/qderiv ==
  w : Inport
  q : Inport  Port=2
  Mux : Mux  Inputs=2
  Mux1 : Mux
  qd1 : Fcn  Expr=(u(7)*u(1)-u(6)*u(2)+u(5)*u(3))/2
  qd2 : Fcn  Expr=(u(6)*u(1)+u(7)*u(2)-u(4)*u(3))/2
  qd3 : Fcn  Expr=(-u(5)*u(1)+u(4)*u(2)+u(7)*u(3))/2
  qd4 : Fcn  Expr=(-u(4)*u(1)-u(5)*u(2)-u(6)*u(3))/2
  qd : Outport
  wires:
  w/1 -> Mux/1
  q/1 -> Mux/2
  Mux/1 -> qd3/1, qd4/1, qd1/1, qd2/1
  qd1/1 -> Mux1/1
  qd2/1 -> Mux1/2
  qd3/1 -> Mux1/3
  qd4/1 -> Mux1/4
  Mux1/1 -> qd/1

== system top_model_rw_desatTest/Controller1/Free Rigid Body with Momentum Actuators2/RWA Saturation Model (Maxon EC 32 Flat 15W 24V)/max rate check ==
  wheel h : Inport
  wheel hb : Inport  Port=2
  0 to 1 : Constant  Value=0  VectorParams1D=off
  "0 to 1 " : Constant  Value=0  VectorParams1D=off
  "0 to 1  " : Constant  Value=0  VectorParams1D=off
  Abs : Abs  SaturateOnIntegerOverflow=on
  Demux : Demux  Outputs=3
  Demux1 : Demux  Outputs=3
  Demux2 : Demux  Outputs=3
  Logical Operator : Logic
  Logical Operator1 : Logic
  Logical Operator2 : Logic
  Mux : Mux  Inputs=3
  Product : Product  SaturateOnIntegerOverflow=on  InputSameDT=on  OutDataTypeStr=Inherit: Same as first input
  Product1 : Product  SaturateOnIntegerOverflow=on  InputSameDT=on  OutDataTypeStr=Inherit: Same as first input
  Product2 : Product  SaturateOnIntegerOverflow=on  InputSameDT=on  OutDataTypeStr=Inherit: Same as first input
  Relational Operator : RelationalOperator  RndMeth=Nearest  InputSameDT=on
  Relational Operator1 : RelationalOperator  RndMeth=Nearest  InputSameDT=on
  Relational Operator2 : RelationalOperator  RndMeth=Nearest  InputSameDT=on
  Sign{,1..5} (6 alike) : Signum
  gt : RelationalOperator  Operator=>  RndMeth=Nearest  InputSameDT=on
  "gt " : RelationalOperator  Operator=>  RndMeth=Nearest  InputSameDT=on
  "gt  " : RelationalOperator  Operator=>  RndMeth=Nearest  InputSameDT=on
  hmax : Constant  Value=hmax  VectorParams1D=off
  hmax1 : Constant  Value=hmax  VectorParams1D=off
  hmax2 : Constant  Value=hmax  VectorParams1D=off
  saturated? : Outport
  wires:
  Abs/1 -> Demux/1
  Demux/1 -> Relational Operator/1
  Demux/2 -> Relational Operator1/1
  Demux/3 -> Relational Operator2/1
  hmax/1 -> Relational Operator/2
  hmax1/1 -> Relational Operator1/2
  hmax2/1 -> Relational Operator2/2
  wheel h/1 -> Abs/1, Demux2/1
  Mux/1 -> saturated?/1
  wheel hb/1 -> Demux1/1
  Demux1/1 -> Sign3/1
  Demux1/2 -> Sign4/1
  Demux1/3 -> Sign5/1
  Sign/1 -> Product/1
  Sign3/1 -> Product/2
  Sign1/1 -> Product1/1
  Sign4/1 -> Product1/2
  Sign2/1 -> Product2/1
  Sign5/1 -> Product2/2
  0 to 1/1 -> gt/2
  Product/1 -> gt/1
  "0 to 1 "/1 -> "gt "/2
  Product1/1 -> "gt "/1
  "0 to 1  "/1 -> "gt  "/2
  Product2/1 -> "gt  "/1
  Logical Operator/1 -> Mux/1
  Logical Operator1/1 -> Mux/2
  Logical Operator2/1 -> Mux/3
  Relational Operator/1 -> Logical Operator/1
  Relational Operator1/1 -> Logical Operator1/1
  Relational Operator2/1 -> Logical Operator2/1
  gt/1 -> Logical Operator/2
  "gt "/1 -> Logical Operator1/2
  "gt  "/1 -> Logical Operator2/2
  Demux2/1 -> Sign/1
  Demux2/2 -> Sign1/1
  Demux2/3 -> Sign2/1

== system top_model_rw_desatTest/Controller1/Free Rigid Body with Momentum Actuators2/compute attitude error/quat_multiply (relative quat) ==
  q_bc : Inport
  q_ab : Inport  Port=2
  Mux : Mux  Inputs=2
  Mux1 : Mux
  qerr1 : Fcn  Expr=u(4)*u(5)+u(3)*u(6)-u(2)*u(7)+u(1)*u(8)
  qerr2 : Fcn  Expr=-u(3)*u(5)+u(4)*u(6)+u(1)*u(7)+u(2)*u(8)
  qerr3 : Fcn  Expr=u(2)*u(5)-u(1)*u(6)+u(4)*u(7)+u(3)*u(8)
  qerr4 : Fcn  Expr=-u(1)*u(5)-u(2)*u(6)-u(3)*u(7)+u(4)*u(8)
  q_ac : Outport
  wires:
  Mux1/1 -> q_ac/1
  qerr4/1 -> Mux1/4
  qerr3/1 -> Mux1/3
  qerr2/1 -> Mux1/2
  qerr1/1 -> Mux1/1
  Mux/1 -> qerr4/1, qerr3/1, qerr2/1, qerr1/1
  q_ab/1 -> Mux/2
  q_bc/1 -> Mux/1

== system top_model_rw_desatTest/Controller1/Normal Mode Control System/compute attitude error/quat_multiply (relative quat) ==
  q_bc : Inport
  q_ab : Inport  Port=2
  Mux : Mux  Inputs=2
  Mux1 : Mux
  qerr1 : Fcn  Expr=u(4)*u(5)+u(3)*u(6)-u(2)*u(7)+u(1)*u(8)
  qerr2 : Fcn  Expr=-u(3)*u(5)+u(4)*u(6)+u(1)*u(7)+u(2)*u(8)
  qerr3 : Fcn  Expr=u(2)*u(5)-u(1)*u(6)+u(4)*u(7)+u(3)*u(8)
  qerr4 : Fcn  Expr=-u(1)*u(5)-u(2)*u(6)-u(3)*u(7)+u(4)*u(8)
  q_ac : Outport
  wires:
  Mux1/1 -> q_ac/1
  qerr4/1 -> Mux1/4
  qerr3/1 -> Mux1/3
  qerr2/1 -> Mux1/2
  qerr1/1 -> Mux1/1
  Mux/1 -> qerr4/1, qerr3/1, qerr2/1, qerr1/1
  q_ab/1 -> Mux/2
  q_bc/1 -> Mux/1

== system top_model_rw_desatTest/Controller1/Normal Mode Control System/compute attitude error/quat_multiply (relative quat)1 ==
  q_bc : Inport
  q_ab : Inport  Port=2
  Mux : Mux  Inputs=2
  Mux1 : Mux
  qerr1 : Fcn  Expr=u(4)*u(5)+u(3)*u(6)-u(2)*u(7)+u(1)*u(8)
  qerr2 : Fcn  Expr=-u(3)*u(5)+u(4)*u(6)+u(1)*u(7)+u(2)*u(8)
  qerr3 : Fcn  Expr=u(2)*u(5)-u(1)*u(6)+u(4)*u(7)+u(3)*u(8)
  qerr4 : Fcn  Expr=-u(1)*u(5)-u(2)*u(6)-u(3)*u(7)+u(4)*u(8)
  q_ac : Outport
  wires:
  Mux1/1 -> q_ac/1
  qerr4/1 -> Mux1/4
  qerr3/1 -> Mux1/3
  qerr2/1 -> Mux1/2
  qerr1/1 -> Mux1/1
  Mux/1 -> qerr4/1, qerr3/1, qerr2/1, qerr1/1
  q_ab/1 -> Mux/2
  q_bc/1 -> Mux/1

== system top_model_rw_desatTest/Controller1/Propulsion/Subsystem/Activation ==
  note: current time
  note: time of trigger
  note: t_trig + onTime
  hit : Inport
  T_maneuver : Inport  Port=2
  Add : Sum
  Clock : Clock
  Hit Crossing : HitCross
  Subsystem : Subsystem
  Subtract : Sum  Inputs=+-
  man_end : Outport
  wires:
  Clock/1 -> Subsystem/1(input), Subtract/1
  hit/1 -> Subsystem/2(overwrite trigger)
  Hit Crossing/1 -> man_end/1
  T_maneuver/1 -> Add/2
  Subsystem/1(value) -> Add/1
  Add/1 -> Subtract/2
  Subtract/1 -> Hit Crossing/1

== system top_model_rw_desatTest/Controller1/Propulsion/Subsystem/Subsystem ==
  input : Inport
  overwrite trigger : Inport  Port=2
  Data Store Memory : DataStoreMemory  DataStoreName=Mem  ShowAdditionalParam=off
  Data Store Read : DataStoreRead  DataStoreName=Mem  SampleTime=[0,0]  DataStoreElements=Mem
  Data Store Write : DataStoreWrite  DataStoreName=Mem  SampleTime=[0,0]  DataStoreElements=Mem
  Switch : Switch  Criteria=u2 > Threshold
  value : Outport
  wires:
  input/1 -> Switch/1
  Switch/1 -> Data Store Write/1, value/1
  Data Store Read/1 -> Switch/3
  overwrite trigger/1 -> Switch/2

== system top_model_rw_desatTest/GNC/Follower Maneuver/Optimal Latitude Calc/Enabled Subsystem ==
  r : Inport
  v : Inport  Port=2
  x_tgt : Inport  Port=3
  x_f : Inport  Port=4
  K : Inport  Port=5
  L : Inport  Port=6
  "muE " : Inport  Port=7
  Enable : EnablePort
  MATLAB Function : MATLAB Function  TreatAsAtomicUnit=on
  dV_opt : Outport
  long_opt : Outport  Port=2
  pos_opt : Outport  Port=3
  wires:
  r/1 -> MATLAB Function/1(r)
  v/1 -> MATLAB Function/2(v)
  "muE "/1 -> MATLAB Function/7(muE)
  x_tgt/1 -> MATLAB Function/3(x_t)
  x_f/1 -> MATLAB Function/4(x)
  K/1 -> MATLAB Function/5(K)
  L/1 -> MATLAB Function/6(L)
  MATLAB Function/3(long_opt) -> long_opt/1
  MATLAB Function/1(dV_opt) -> dV_opt/1
  MATLAB Function/2(pos_opt) -> pos_opt/1

== system top_model_rw_desatTest/Controller/Propulsion/Subsystem/Activation/Subsystem ==
  input : Inport
  overwrite trigger : Inport  Port=2
  Data Store Memory : DataStoreMemory  DataStoreName=Mem  ShowAdditionalParam=off
  Data Store Read : DataStoreRead  DataStoreName=Mem  SampleTime=[0,0]  DataStoreElements=Mem
  Data Store Write : DataStoreWrite  DataStoreName=Mem  SampleTime=[0,0]  DataStoreElements=Mem
  Switch : Switch  Criteria=u2 > Threshold
  value : Outport
  wires:
  input/1 -> Switch/1
  Switch/1 -> value/1, Data Store Write/1
  Data Store Read/1 -> Switch/3
  overwrite trigger/1 -> Switch/2

== system top_model_rw_desatTest/Controller1/Propulsion/Subsystem/Activation/Subsystem ==
  input : Inport
  overwrite trigger : Inport  Port=2
  Data Store Memory : DataStoreMemory  DataStoreName=Mem  ShowAdditionalParam=off
  Data Store Read : DataStoreRead  DataStoreName=Mem  SampleTime=[0,0]  DataStoreElements=Mem
  Data Store Write : DataStoreWrite  DataStoreName=Mem  SampleTime=[0,0]  DataStoreElements=Mem
  Switch : Switch  Criteria=u2 > Threshold
  value : Outport
  wires:
  input/1 -> Switch/1
  Switch/1 -> value/1, Data Store Write/1
  Data Store Read/1 -> Switch/3
  overwrite trigger/1 -> Switch/2

== matlab function top_model_rw_desatTest/Attitude Determination and Desired Attitude1/Attitude Determination/Generate reference vectors from Ephemeris and Magnetic Field Model/DecimalYearIncrement/MATLAB Function ==
  data: DecimalYear output; year input; month input; day input; hour input; minute input; second input
function DecimalYear = fcn(year,month,day,hour,minute,second)

for i=1:month-1
    if (month == 1 || month == 3 || month == 5 || month == 7 ...
             || month == 8 || month == 10 || month == 12)
         day= day+31;
    elseif (month == 2)
        if isLeapYear(year)
            day= day+29;
        else
            day= day+28;
        end
    else
        day= day+30;
    end
end
DecimalYear= year ...
            +day/(365+isLeapYear(year))   ...
            +hour/(365+isLeapYear(year))/24 ...
            +minute/(365+isLeapYear(year))/24/60 ...
            +second/(365+isLeapYear(year))/24/3600;
end
        
function logical=isLeapYear(year)
if (rem(year,4)==0)
    if (rem(year,100)==0)
        if (rem(year,400)==0)
            logical=1;
        else
            logical=0;
        end
    else
        logical=1;
    end
else
    logical=0;
end
end

== matlab function top_model_rw_desatTest/Attitude Determination and Desired Attitude1/Attitude Determination/Subsystem/MATLAB Function ==
  data: N_sun input; N_mag input; q_triad output; B_sun input; B_mag input
function q_triad = TRIAD(N_sun, N_mag, B_sun, B_mag)
%Based on time and the location of the spacecraft, the sun and magnetic 
%field vectors in the reference frame N are provided. Based on the sun
%sensor and magnetometer readings, the sun and magnetic field vectors are
%provided in the spacecraft's body frame B. This TRIAD algorithm is very
%straightforward and will not be used on the spacecraft, only for the
%sumulation. B/c the algorithm has the orientation of the same vectors in
%different reference frame, it is able to compute the rotation between
%those reference frames. The algorithm will fail if either of the reference
%vectors or observed vectors are parallel or anti parallel.

% Normalize all vectors (should be normalized already)
N_sun=N_sun/norm(N_sun);
B_sun=B_sun/norm(B_sun);
N_mag=N_mag/norm(N_mag);
B_mag=B_mag/norm(B_mag);

% Ensure all vectors have three components and vectors in the same frame
% are not parallel
if size(N_sun)~=[3 1]
    error('N_sun must be a 3-component column vector')
end

if size(B_sun)~=[3 1]
    error('B_sun must be a 3-component column vector')
end

if size(N_mag)~=[3 1]
    error('N_mag must be a 3-component column vector')
end

if size(B_mag)~=[3 1]
    error('B_mag must be a 3-component column vector')
end

if dot(N_sun,N_mag)==1
    error('Reference frame N vectors can not be parallel')
end

if dot(B_sun,B_mag)==1
    error('Body frame B vectors can not be parallel')
end

% Compute orthonogoal right-handed vectors of reference frame
v1=N_sun;
v2=cross(N_sun,N_mag)/norm(cross(N_sun,N_mag));
v3=cross(v1,v2);

% Compute orthonogoal right-handed vectors of body frame
w1=B_sun;
w2=cross(B_sun,B_mag)/norm(cross(B_sun,B_mag));
w3=cross(w1,w2);

DCM_be=w1(:)*v1(:)'+w3(:)*v3(:)'+w2(:)*v2(:)';
tr= DCM_be(1,1) + DCM_be(2,2) + DCM_be(3,3);
th= acos((tr-1)/2);
axis= 0.5/sin(th)*[DCM_be(2,3)-DCM_be(3,2);DCM_be(3,1)-DCM_be(1,3);DCM_be(1,2)-DCM_be(2,1)];
q_triad= [axis*sin(th/2);cos(th/2)];
%q_triad=dcm2quat(DCM_triad);
% q_temp=DCM_triad;
% q_triad=[q_temp(2) q_temp(3) q_temp(4) q_temp(1)];
end

== matlab function top_model_rw_desatTest/Attitude Determination and Desired Attitude/Attitude Determination/Generate reference vectors from Ephemeris and Magnetic Field Model/DecimalYearIncrement/MATLAB Function ==
  data: DecimalYear output; year input; month input; day input; hour input; minute input; second input
function DecimalYear = fcn(year,month,day,hour,minute,second)

for i=1:month-1
    if (month == 1 || month == 3 || month == 5 || month == 7 ...
             || month == 8 || month == 10 || month == 12)
         day= day+31;
    elseif (month == 2)
        if isLeapYear(year)
            day= day+29;
        else
            day= day+28;
        end
    else
        day= day+30;
    end
end
DecimalYear= year ...
            +day/(365+isLeapYear(year))   ...
            +hour/(365+isLeapYear(year))/24 ...
            +minute/(365+isLeapYear(year))/24/60 ...
            +second/(365+isLeapYear(year))/24/3600;
end
        
function logical=isLeapYear(year)
if (rem(year,4)==0)
    if (rem(year,100)==0)
        if (rem(year,400)==0)
            logical=1;
        else
            logical=0;
        end
    else
        logical=1;
    end
else
    logical=0;
end
end

== matlab function top_model_rw_desatTest/GNC/Follower Maneuver/Impulse Conversion ==
  data: dV_raw input; m_follower input; Imp_filt output; Imp_max input; Imp_min input
function Imp_filt = fcn(dV_raw,m_follower,Imp_max,Imp_min)
%#codegen

Imp_raw = dV_raw*m_follower;

if (norm(Imp_raw)>Imp_max)
    Imp_red=Imp_raw*(Imp_max/norm(Imp_raw));
elseif (norm(Imp_raw)<Imp_min)
    Imp_red=[0;0;0];
else
    Imp_red=Imp_raw;
end

Imp_filt = Imp_red;

== matlab function top_model_rw_desatTest/GNC/Follower Maneuver/Optimal Latitude Calc/Enabled Subsystem/MATLAB Function ==
  data: dV_opt output; pos_opt output; long_opt output; r input; v input; x_t input; x input; K input; L input; muE input
function [dV_opt,pos_opt,long_opt] = fcn(r,v,x_t,x,K,L,muE)
%#codegen

z0=[r;v];

E=norm(v)^2/2-muE/norm(r);
a=-muE/(2*E);
T=2*pi/sqrt(muE)*a^(3/2);

options=odeset('AbsTol',1e-12,'RelTol',1e-12);
tspan=linspace(0,T,10000);
[~,zs] = ode45(@orbit1diff,tspan,z0,options,muE,[0;0;0]);

dV_opt = [0;0;0];
pos_opt = [0;0;0];
max_rat=0;
rat=0;
long_opt=0;
N=length(tspan);
x_f=x;
x_diff=x_t-x_f;
% x_diff_hat=x_diff/norm(x_diff);

for i=1:N
    r_f=zs(i,1:3);
    v_f=zs(i,4:6);
    
%     if (abs(dot(r_f,v_f))<perpTol)
%         rat=-999999;
%     end
    
    A=[crs(r_f);
       v_f];

    B=(crs(v_f)*crs(r_f)-crs(crs(r_f)*v_f'))/muE;    
    M=[A;
       B];

    dV_vec=pinv(M)*x_diff;
    dV_opt_sqd=dV_vec'*L*dV_vec;
    dx_vec=M*dV_vec;
    dx_opt_sqd=dx_vec'*K*dx_vec;
    
    rat=dx_opt_sqd/dV_opt_sqd;
    
    if (rat>max_rat)
        max_rat = rat;
        long_opt = atan2(r_f(2),r_f(1));
        pos_opt = r_f';
        dV_opt = dV_vec;
        if (long_opt<0)
            long_opt=long_opt+2*pi;
        end
    end
end
end

== matlab function top_model_rw_desatTest/Attitude Determination and Desired Attitude/Position and Velocity to Desired Attitude in Quat/dcm2quat ==
  data: DCM_be input; q output; tr output; q_prev input; flag output
function [q, tr, flag] = fcn(DCM_be,q_prev)
tr= DCM_be(1,1) + DCM_be(2,2) + DCM_be(3,3);
flag=[0 1];
if (tr > 0)
    S= sqrt(1+tr)*2;
    q4= 0.25 * S;
    q1= (DCM_be(3,2)-DCM_be(2,3))/S;
    q2= (DCM_be(1,3)-DCM_be(3,1))/S;
    q3= (DCM_be(2,1)-DCM_be(1,2))/S;
    q=[q1;q2;q3;q4];
    flag(1)=1;
    
elseif ((DCM_be(1,1)>DCM_be(2,2)) && (DCM_be(1,1)>DCM_be(3,3)))
    S= sqrt(1+DCM_be(1,1)-DCM_be(2,2)-DCM_be(3,3))*2;
    q4= (DCM_be(3,2)-DCM_be(2,3))/S;
    q1= 0.25*S;
    q2= (DCM_be(1,2)+DCM_be(2,1))/S;
    q3= (DCM_be(1,3)+DCM_be(3,1))/S;
    flag(1)=2;
    q=[q1;q2;q3;q4];
elseif (DCM_be(2,2)>DCM_be(3,3))
    S= sqrt(1+DCM_be(2,2)-DCM_be(1,1)-DCM_be(3,3))*2;
    q4= (DCM_be(1,3)-DCM_be(3,1))/S;
    q1= (DCM_be(1,2)+DCM_be(2,1))/S;
    q2= 0.25*S;
    q3= (DCM_be(2,3)+DCM_be(3,2))/S;
    flag(1)=3;
    q=[q1;q2;q3;q4];
else
    S= sqrt(1+DCM_be(3,3)-DCM_be(1,1)-DCM_be(2,2))*2;
    q4= (DCM_be(2,1)-DCM_be(1,2))/S;
    q1= (DCM_be(1,3)+DCM_be(3,1))/S;
    q2= (DCM_be(2,3)+DCM_be(3,2))/S;
    q3= 0.25*S;
    flag(1)=4;
    q=[q1;q2;q3;q4];
end


if  (flag(2)*sign(q(1))*sign(q_prev(1))==-1 && q(1)*q(1)>1e-8) || ...
    (flag(2)*sign(q(2))*sign(q_prev(2))==-1 && q(2)*q(2)>1e-8) || ...
    (flag(2)*sign(q(3))*sign(q_prev(3))==-1 && q(3)*q(3)>1e-8)
    %sign(q_prev(1))==0 || ...
    %sign(q_prev(2))==0 || ...
    %sign(q_prev(3))==0
    
    flag(2)=flag(2)*-1;
end
if flag(2)==-1
    q=-q;
end

== matlab function top_model_rw_desatTest/LDR_Plant/Atmospheric drag ==
  data: velocity input; drag output
function drag = fcn(velocity)
V= norm(velocity);    % 
A= 0.01*0.01;   % 10cm x 10cm
Cd= 0.82;       % for long square cylinder
drag = Cd * A * .5 * 1e-8 * V * -velocity;
